simulink model "FAdder"  (R2014a)
settings: Solver=ode45  StartTime=0.0  StopTime=10.0  RelTol=1e-3
settings Model: Creator=Shiyu  LastModifiedBy=Shiyu

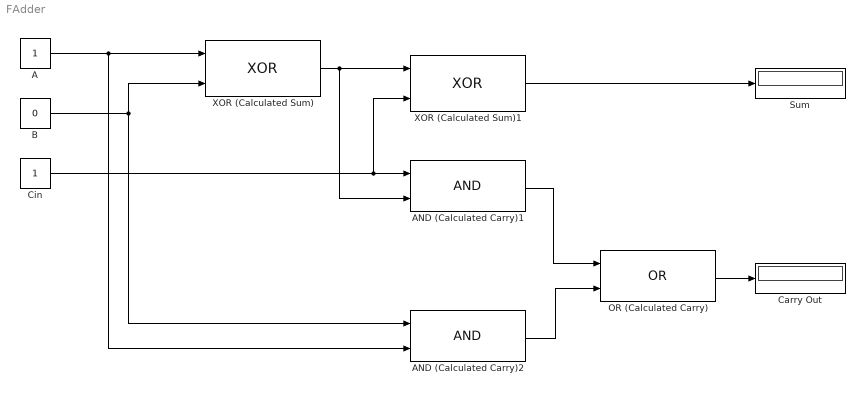
== system FAdder ==
  A : Constant
  AND (Calculated Carry)1 : Logic  AllPortsSameDT=off  OutDataTypeStr=boolean
  AND (Calculated Carry)2 : Logic  AllPortsSameDT=off  OutDataTypeStr=boolean
  B : Constant  Value=0
  Carry Out : Display
  Cin : Constant
  OR (Calculated Carry) : Logic  Operator=OR  AllPortsSameDT=off  OutDataTypeStr=boolean
  Sum : Display
  XOR (Calculated Sum) : Logic  Operator=XOR  AllPortsSameDT=off  OutDataTypeStr=boolean
  XOR (Calculated Sum)1 : Logic  Operator=XOR  AllPortsSameDT=off  OutDataTypeStr=boolean
  wires:
  A/1 -> AND (Calculated Carry)2/2, XOR (Calculated Sum)/1
  B/1 -> AND (Calculated Carry)2/1, XOR (Calculated Sum)/2
  XOR (Calculated Sum)/1 -> AND (Calculated Carry)1/2, XOR (Calculated Sum)1/1
  OR (Calculated Carry)/1 -> Carry Out/1
  XOR (Calculated Sum)1/1 -> Sum/1
  Cin/1 -> XOR (Calculated Sum)1/2, AND (Calculated Carry)1/1
  AND (Calculated Carry)1/1 -> OR (Calculated Carry)/1
  AND (Calculated Carry)2/1 -> OR (Calculated Carry)/2
